simulink model "PID_ADRC_v2"  (R2022a)
settings: Solver=VariableStepAuto  StartTime=0.0  StopTime=10.0  RelTol=1e-3
libraries: slpidlib x2
settings Model: Creator=ducdu  LastModifiedBy=ducdu
settings DebuggingCC: UnderSpecifiedDimensionMsg=warning

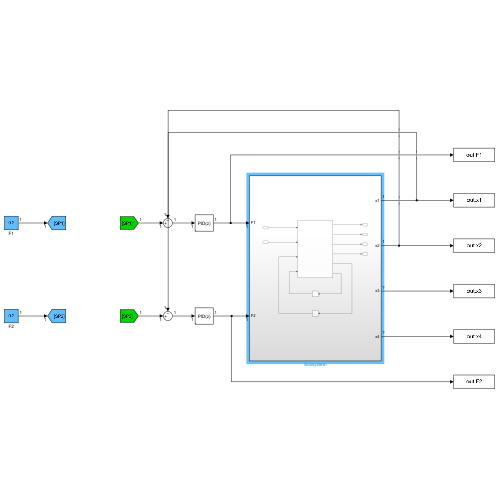
[thumbnail: Simulink's stored preview of the top-level diagram]
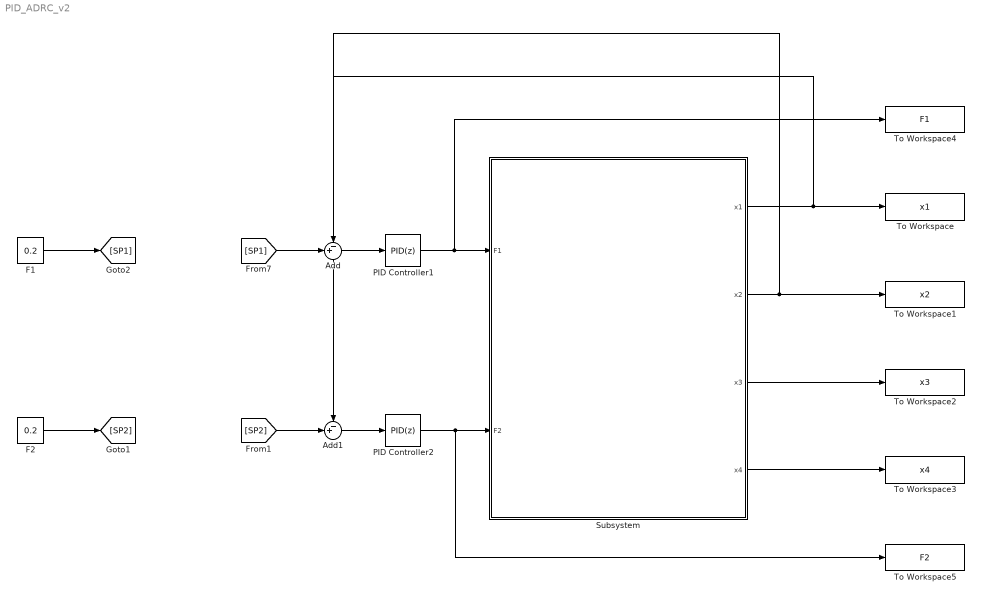
== system PID_ADRC_v2 ==
  Add : Sum  Inputs=-+|
  Add1 : Sum  Inputs=-+|
  F1 : Constant  Value=0.2
  F2 : Constant  Value=0.2
  PID Controller1 : slpidlib/PID Controller  Controller=PID  Form=Parallel  TimeDomain=Discrete-time  UseExternalTs=off  SampleTime=0.003  IntegratorMethod=Forward Euler  FilterMethod=Forward Euler  ControllerParametersSource=internal  P=0.18380080341484  I=0.00264427661684036  UseKiTs=off  D=14.3583596221209  N=105.481990683281  UseFilter=on  TunerSelectOption=Transfer Function Based (PID Tuner App)  InitialConditionSource=internal  InitialConditionForIntegrator=0  InitialConditionForFilter=0  DifferentiatorICPrevScaledInput=0  ExternalReset=none  TrackingMode=off  Kt=1  LimitOutput=off  SatLimitsSource=internal  UpperSaturationLimit=inf  LowerSaturationLimit=-inf  LinearizeAsGain=on  AntiWindupMode=none  Kb=1  POutMin=[]  POutMax=[]  IOutMin=[]  IOutMax=[]  DOutMin=[]  DOutMax=[]  NOutMin=[]  NOutMax=[]  SumOutMin=[]  SumOutMax=[]  SaturationOutMin=[]  SaturationOutMax=[]  PParamMin=[]  PParamMax=[]  IParamMin=[]  IParamMax=[]  DParamMin=[]  DParamMax=[]  NParamMin=[]  NParamMax=[]  KbParamMin=[]  KbParamMax=[]  KtParamMin=[]  KtParamMax=[]  KbOutMin=[]  KbOutMax=[]  KtOutMin=[]  KtOutMax=[]  IntegratorOutMin=[]  IntegratorOutMax=[]  FilterOutMin=[]  FilterOutMax=[]  SumI1OutMin=[]  SumI1OutMax=[]  SumI2OutMin=[]  SumI2OutMax=[]  SumI3OutMin=[]  SumI3OutMax=[]  SumI4OutMin=[]  SumI4OutMax=[]  SumDOutMin=[]  SumDOutMax=[]  DifferentiatorOutMin=[]  DifferentiatorOutMax=[]  FilterDiffOutCoefMin=[]  FilterDiffOutCoefMax=[]  ReciprocalOutMin=[]  ReciprocalOutMax=[]  SumDenOutMin=[]  SumDenOutMax=[]  SumNumOutMin=[]  SumNumOutMax=[]  DivideOutMin=[]  DivideOutMax=[]  UdiffTsProdOutMin=[]  UdiffTsProdOutMax=[]  NTsProdOutMin=[]  NTsProdOutMax=[]  UintegralTsProdOutMin=[]  UintegralTsProdOutMax=[]  UngainTsProdOutMin=[]  UngainTsProdOutMax=[]  IntegratorContinuousStateAttributes=''  IntegratorStateMustResolveToSignalObject=off  IntegratorRTWStateStorageClass=Auto  FilterContinuousStateAttributes=''  FilterStateMustResolveToSignalObject=off  FilterRTWStateStorageClass=Auto  ParallelPVariant=InternalParameters  IdealPVariant=Disabled  IVariant=InternalParameters  DVariant=InternalParameters  IntegratorVariant=Discrete  SatVariant=Disabled  AWVariant=Passthrough  PCopyVariant=Disabled  TRVariant=Disabled  FdbkBlocksVariant=Forward  IdealPFdbkVariant=Disabled  SatFdbkVariant=Disabled  DerivativeFilterVariant=ForwardEulerFilter  NVariant=InternalParameters  NCopyVariant=Disabled  FilterICVariant=InternalICsFilter  IntegratorICVariant=InternalICs  ExternalResetVariant=Disabled  TRSumVariant=Passthrough  SumFdbkVariant=Disabled  SumVariant=Sum_PID  TsampFilterVariant=InternalTs  TsampNgainVariant=Passthrough  TsampIntegralVariant=Passthrough  ExternalSaturationOutDataTypeStr=Inherit: Same as second input  aMode=0
  PID Controller2 : slpidlib/PID Controller  Controller=PID  Form=Parallel  TimeDomain=Discrete-time  UseExternalTs=off  SampleTime=0.003  IntegratorMethod=Forward Euler  FilterMethod=Forward Euler  ControllerParametersSource=internal  P=0.18380080341484  I=0.00264427661684036  UseKiTs=off  D=14.3583596221209  N=105.481990683281  UseFilter=on  TunerSelectOption=Transfer Function Based (PID Tuner App)  InitialConditionSource=internal  InitialConditionForIntegrator=0  InitialConditionForFilter=0  DifferentiatorICPrevScaledInput=0  ExternalReset=none  TrackingMode=off  Kt=1  LimitOutput=off  SatLimitsSource=internal  UpperSaturationLimit=inf  LowerSaturationLimit=-inf  LinearizeAsGain=on  AntiWindupMode=none  Kb=1  POutMin=[]  POutMax=[]  IOutMin=[]  IOutMax=[]  DOutMin=[]  DOutMax=[]  NOutMin=[]  NOutMax=[]  SumOutMin=[]  SumOutMax=[]  SaturationOutMin=[]  SaturationOutMax=[]  PParamMin=[]  PParamMax=[]  IParamMin=[]  IParamMax=[]  DParamMin=[]  DParamMax=[]  NParamMin=[]  NParamMax=[]  KbParamMin=[]  KbParamMax=[]  KtParamMin=[]  KtParamMax=[]  KbOutMin=[]  KbOutMax=[]  KtOutMin=[]  KtOutMax=[]  IntegratorOutMin=[]  IntegratorOutMax=[]  FilterOutMin=[]  FilterOutMax=[]  SumI1OutMin=[]  SumI1OutMax=[]  SumI2OutMin=[]  SumI2OutMax=[]  SumI3OutMin=[]  SumI3OutMax=[]  SumI4OutMin=[]  SumI4OutMax=[]  SumDOutMin=[]  SumDOutMax=[]  DifferentiatorOutMin=[]  DifferentiatorOutMax=[]  FilterDiffOutCoefMin=[]  FilterDiffOutCoefMax=[]  ReciprocalOutMin=[]  ReciprocalOutMax=[]  SumDenOutMin=[]  SumDenOutMax=[]  SumNumOutMin=[]  SumNumOutMax=[]  DivideOutMin=[]  DivideOutMax=[]  UdiffTsProdOutMin=[]  UdiffTsProdOutMax=[]  NTsProdOutMin=[]  NTsProdOutMax=[]  UintegralTsProdOutMin=[]  UintegralTsProdOutMax=[]  UngainTsProdOutMin=[]  UngainTsProdOutMax=[]  IntegratorContinuousStateAttributes=''  IntegratorStateMustResolveToSignalObject=off  IntegratorRTWStateStorageClass=Auto  FilterContinuousStateAttributes=''  FilterStateMustResolveToSignalObject=off  FilterRTWStateStorageClass=Auto  ParallelPVariant=InternalParameters  IdealPVariant=Disabled  IVariant=InternalParameters  DVariant=InternalParameters  IntegratorVariant=Discrete  SatVariant=Disabled  AWVariant=Passthrough  PCopyVariant=Disabled  TRVariant=Disabled  FdbkBlocksVariant=Forward  IdealPFdbkVariant=Disabled  SatFdbkVariant=Disabled  DerivativeFilterVariant=ForwardEulerFilter  NVariant=InternalParameters  NCopyVariant=Disabled  FilterICVariant=InternalICsFilter  IntegratorICVariant=InternalICs  ExternalResetVariant=Disabled  TRSumVariant=Passthrough  SumFdbkVariant=Disabled  SumVariant=Sum_PID  TsampFilterVariant=InternalTs  TsampNgainVariant=Passthrough  TsampIntegralVariant=Passthrough  ExternalSaturationOutDataTypeStr=Inherit: Same as second input  aMode=0
  Subsystem : Subsystem
  To Workspace : ToWorkspace  VariableName=x1  SaveFormat=Timeseries  SampleTime=-1
  To Workspace1 : ToWorkspace  VariableName=x2  SaveFormat=Timeseries  SampleTime=-1
  To Workspace2 : ToWorkspace  VariableName=x3  SaveFormat=Timeseries  SampleTime=-1
  To Workspace3 : ToWorkspace  VariableName=x4  SaveFormat=Timeseries  SampleTime=-1
  To Workspace4 : ToWorkspace  VariableName=F1  SaveFormat=Timeseries  SampleTime=-1
  To Workspace5 : ToWorkspace  VariableName=F2  SaveFormat=Timeseries  SampleTime=-1
  wires:
  F1/1 -> [SP1]
  [SP1] -> Add/2
  PID Controller1/1 -> To Workspace4/1, Subsystem/1(F1)
  Add/1 -> PID Controller1/1
  F2/1 -> [SP2]
  [SP2] -> Add1/2
  Add1/1 -> PID Controller2/1
  PID Controller2/1 -> To Workspace5/1, Subsystem/2(F2)
  Subsystem/1(x1) -> To Workspace/1, Add/1
  Subsystem/2(x2) -> To Workspace1/1, Add1/1
  Subsystem/3(x3) -> To Workspace2/1
  Subsystem/4(x4) -> To Workspace3/1

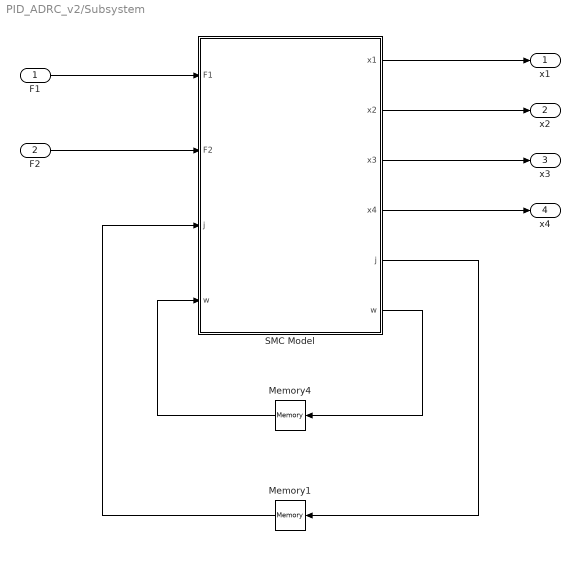
== system PID_ADRC_v2/Subsystem ==
  F1 : Inport
  F2 : Inport  Port=2
  Memory1 : Memory
  Memory4 : Memory  InitialCondition=zeros(20,20000)
  SMC Model : MATLAB Function  TreatAsAtomicUnit=on
  x1 : Outport
  x2 : Outport  Port=2
  x3 : Outport  Port=3
  x4 : Outport  Port=4
  wires:
  F1/1 -> SMC Model/1(F1)
  SMC Model/6(w) -> Memory4/1
  Memory1/1 -> SMC Model/3("j ")
  SMC Model/2(x2) -> x2/1
  SMC Model/5(j) -> Memory1/1
  SMC Model/1(x1) -> x1/1
  F2/1 -> SMC Model/2(F2)
  Memory4/1 -> SMC Model/4("w ")
  SMC Model/3(x3) -> x3/1
  SMC Model/4(x4) -> x4/1

== matlab function PID_ADRC_v2/Subsystem/SMC Model ==
  data: F1 input; F2 input; j input; w input; x1 output; x2 output; x3 output; x4 output; j output; w output
function [x1,x2,x3,x4,j,w] = systemModeling(F1,F2,j,w)
    % Thiết lập các thông số cho dầm
    L = 0.63; EI = 0.754; rho_A = .297;
    % Các vật nặng 
    mw = 13.1; mk = 0.04; mh = 0.86; g = 9.81;
    
    % Thiết lập bước sai phân không gian và thời gian
    n = 9; r = 10000;
    tmax = 15;
    delta_Y = L/(n - 1); % Bước không gian
    delta_t = tmax/(r - 1); % Bước thời gian
    
    x3 = zeros(1,r);
    x2 = 2; 
    dx2dt_2 = zeros(1,r);
    dx2dt_2(1:2) = delta_Y;
    j = j + 1;
    
    %--------------------------------------------------------------------------
    wyyy0 = (w(3,j + 1) - 2*w(2,j + 1) + w(1,j + 1))/(2*delta_Y^3);
    S2 = (F1 - EI*wyyy0)/mw;
    w(1,j + 2) = 2*w(1,j + 1) - w(1,j) + delta_t^2*S2; % 5b
    for i = 3:(n - 2)
        % Đạo hàm theo Y
        wyyyy = (w(i + 2,j + 1) - 4*w(i + 1,j + 1) + 6*w(i,j) - 4*w(i - 1,j + 1) + w(i - 2,j + 1));
        S1 = (-EI/(rho_A*delta_Y^4))*wyyyy; 
        S4 = (-EI/(mh*delta_Y^3))*wyyyy;
    
        % Chuyển động của xe nâng
        dx3dt_2 = (x3(j + 2) - 2*x3(j + 1) + x3(j))/(2*delta_t^2);
        wyx2 = (w(x2 + 1,j) - w(x2 - 1,j))/(2*delta_Y^2);
        dx2dt_2(j + 2) = 2*dx2dt_2(j + 1) - dx2dt_2(j) + (F2 - mh*g - mh*dx3dt_2*wyx2)/mh*delta_t^2; % 5c
    
        % Cập nhật vị trí x2
        if dx2dt_2(j + 2) < delta_Y
            x2 = 2;
            dx2dt_2(j + 2) = delta_Y;
        elseif dx2dt_2(j + 2) > L - delta_Y
            x2 = n - 1;
            dx2dt_2(j + 2) = L - delta_Y;
        else
            x2 = ceil(dx2dt_2(j + 2)/delta_Y);
        end
    
        % Độ lắc của thanh
        if dx2dt_2(j + 2) ~= x2
            w(i,j + 2) = 2*w(i,j + 1) - w(i,j) + delta_t^2*S1; % 5a
            x3(j + 2) = w(i,j + 2) - w(1,j + 2);
        else
            w(i,j + 2) = 2*w(i,j + 1) - w(i,j) + delta_t^2*S4; % 5d
            x3(j + 2) = w(i,j + 2) - w(1,j + 2);
        end
    end
    wyyyl = (-2*w(n,j + 1) + 3*w(n - 1,j + 1) - w(n - 2,j + 1))/(2*delta_Y^3);
    S3 = (EI/mk)*wyyyl;
    w(2,j + 2) = w(1,j + 2);
    w(n,j + 2) = 2*w(n,j + 1) - w(n,j) + delta_t^2*S3; % 5e
    w(n - 1,j + 2) = (w(n,j + 2) + w(n - 2,j + 2))/2;
    
    % Đầu ra
    x1 = w(1,j); % Vị trí xe con
    x2 = dx2dt_2(j); % Vị trí xe nâng
    x3 = x3(j); % Độ lắc xe nâng
    x4 = w(n,j) - w(1,j); % Độ lắc đỉnh thanh

end
